simulink library "Dampers_Axle2_Decoupled"  (R2026a)
settings: Solver=VariableStepAuto
libraries: Damper_Element x4, fl_lib x4
Description:
  | Component of Simscape Vehicle Templates Library
  | 
  | Copyright 2018-2026 The MathWorks, Inc.
settings Model: Creator=smiller  LastModifiedBy=smiller

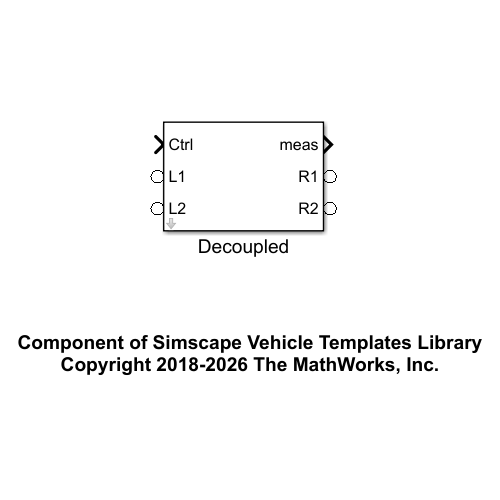
[thumbnail: Simulink's stored preview of the top-level diagram]
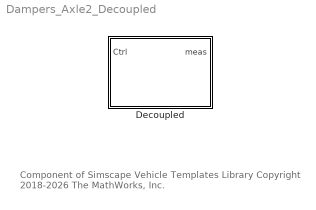
== system Dampers_Axle2_Decoupled ==
  note: Component of Simscape Vehicle Templates Library
      | Copyright 2018-2026 The MathWorks, Inc.
  Decoupled : Subsystem  VariantControl=Independent  mask(Roll and Heave Dampers){}
      mask help: Models dampers in a suspension design that decouples damping for body roll and heave .

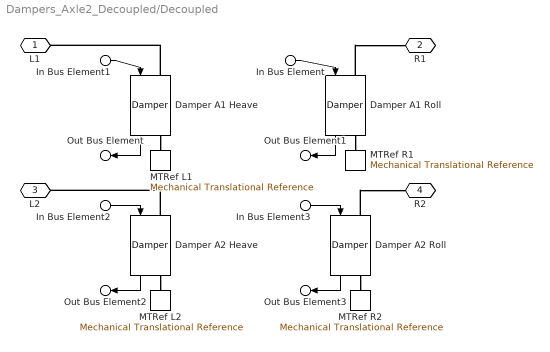
== system Dampers_Axle2_Decoupled/Decoupled ==
  In Bus Element1 : Inport  PortName=Ctrl  Element=L1
  In Bus Element : Inport  PortName=Ctrl  Element=R1
  In Bus Element2 : Inport  PortName=Ctrl  Element=L2
  In Bus Element3 : Inport  PortName=Ctrl  Element=R2
  Damper A1 Heave : Damper_Element/Damper  VariantControl=Variant1  LabelModeActiveChoice=Linear  Damper=Damper.Axle1.Heave  VariantLabel=Damper.Axle1.Heave.class.Value
      settings: AttributesFormatString=%<ActiveVariant>
  Damper A1 Roll : Damper_Element/Damper  VariantControl=Variant1  LabelModeActiveChoice=Linear  Damper=Damper.Axle1.Roll  VariantLabel=Damper.Axle1.Roll.class.Value
      settings: AttributesFormatString=%<ActiveVariant>
  Damper A2 Heave : Damper_Element/Damper  VariantControl=Variant1  LabelModeActiveChoice=Linear  Damper=Damper.Axle2.Heave  VariantLabel=Damper.Axle2.Heave.class.Value
      settings: AttributesFormatString=%<ActiveVariant>
  Damper A2 Roll : Damper_Element/Damper  VariantControl=Variant1  LabelModeActiveChoice=Linear  Damper=Damper.Axle2.Roll  VariantLabel=Damper.Axle2.Roll.class.Value
      settings: AttributesFormatString=%<ActiveVariant>
  MTRef L1 : fl_lib/Mechanical/Translational Elements/Mechanical Translational Reference
  MTRef L2 : fl_lib/Mechanical/Translational Elements/Mechanical Translational Reference
  MTRef R1 : fl_lib/Mechanical/Translational Elements/Mechanical Translational Reference
  MTRef R2 : fl_lib/Mechanical/Translational Elements/Mechanical Translational Reference
  L1 : PMIOPort  Side=Left
  R1 : PMIOPort  Port=2  Side=Right
  L2 : PMIOPort  Port=3  Side=Left
  R2 : PMIOPort  Port=4  Side=Right
  Out Bus Element : Outport  VectorParamsAs1DForOutWhenUnconnected=off  PortName=meas  Element=L1
  Out Bus Element1 : Outport  VectorParamsAs1DForOutWhenUnconnected=off  PortName=meas  Element=R1
  Out Bus Element2 : Outport  VectorParamsAs1DForOutWhenUnconnected=off  PortName=meas  Element=L2
  Out Bus Element3 : Outport  VectorParamsAs1DForOutWhenUnconnected=off  PortName=meas  Element=R2
  wires:
  Damper A2 Roll/1 -> Out Bus Element3/1
  Damper A2 Heave/1 -> Out Bus Element2/1
  In Bus Element2/1 -> Damper A2 Heave/1
  In Bus Element3/1 -> Damper A2 Roll/1
  Damper A1 Roll/1 -> Out Bus Element1/1
  Damper A1 Heave/1 -> Out Bus Element/1
  In Bus Element1/1 -> Damper A1 Heave/1
  In Bus Element/1 -> Damper A1 Roll/1
  connections:
  Damper A1 Heave/RConn1 -- MTRef L1/LConn1
  Damper A1 Heave/LConn1 -- L1/RConn1
  Damper A2 Heave/RConn1 -- MTRef L2/LConn1
  Damper A2 Heave/LConn1 -- L2/RConn1
  Damper A2 Roll/RConn1 -- MTRef R2/LConn1
  Damper A2 Roll/LConn1 -- R2/RConn1
  Damper A1 Roll/RConn1 -- MTRef R1/LConn1
  Damper A1 Roll/LConn1 -- R1/RConn1
